simulink model "X_AXEmodel2"  (R2013b)
settings: Solver=ode45  StartTime=0.0  StopTime=10.0  RelTol=1e-3
libraries: simulink x3, arduinolib x2
settings Model: Creator=KOUSTA  LastModifiedBy=KOUSTA

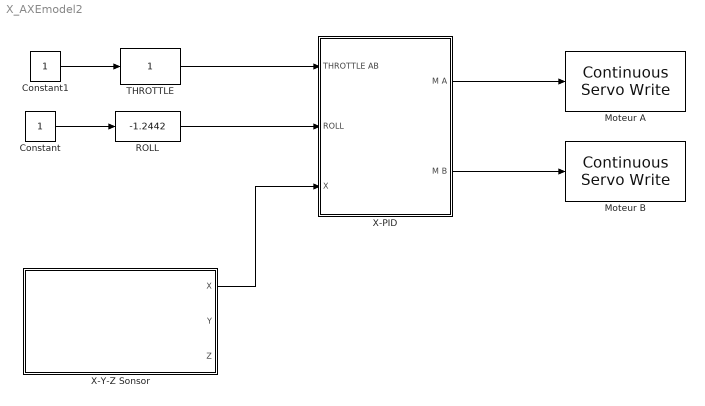
== system X_AXEmodel2 ==
  Constant : Constant
  Constant1 : Constant
  Moteur A : arduinolib/Continuous Servo Write  pinNumber=9
  Moteur B : arduinolib/Continuous Servo Write  pinNumber=3
  ROLL : simulink/Math Operations/Slider Gain  low=-90  gain=-1.2442  high=90
  THROTTLE : simulink/Math Operations/Slider Gain  low=0  gain=1  high=120
  X-PID : Subsystem
  X-Y-Z Sonsor : Subsystem
  wires:
  Constant/1 -> ROLL/1
  Constant1/1 -> THROTTLE/1
  ROLL/1 -> X-PID/2(ROLL)
  X-Y-Z Sonsor/1(X) -> X-PID/3(X)
  X-PID/1(M A) -> Moteur A/1
  X-PID/2(M B) -> Moteur B/1
  THROTTLE/1 -> X-PID/1(THROTTLE AB)

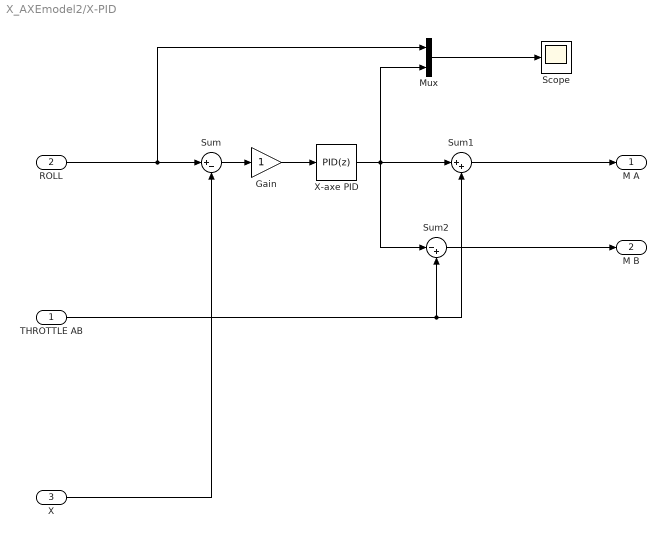
== system X_AXEmodel2/X-PID ==
  THROTTLE AB : Inport
  ROLL : Inport  Port=2
  X : Inport  Port=3
  Gain : Gain
  Mux : Mux  Inputs=2
  Scope : Scope
  Sum : Sum  Inputs=|+-
  Sum1 : Sum  Inputs=|++
  Sum2 : Sum  Inputs=|-+
  X-axe PID : simulink/Continuous/PID Controller  Controller=PID  TimeDomain=Discrete-time  SampleTime=1  IntegratorMethod=Forward Euler  FilterMethod=Forward Euler  Form=Parallel  P=1  I=1  D=0  N=100  InitialConditionSource=internal  InitialConditionForIntegrator=0  InitialConditionForFilter=0  ExternalReset=none  LimitOutput=off  UpperSaturationLimit=inf  LowerSaturationLimit=-inf  LinearizeAsGain=off  AntiWindupMode=none  Kb=1  TrackingMode=off  Kt=1  PParamMin=[]  PParamMax=[]  IParamMin=[]  IParamMax=[]  DParamMin=[]  DParamMax=[]  NParamMin=[]  NParamMax=[]  KbParamMin=[]  KbParamMax=[]  KtParamMin=[]  KtParamMax=[]  POutMin=[]  POutMax=[]  IOutMin=[]  IOutMax=[]  DOutMin=[]  DOutMax=[]  NOutMin=[]  NOutMax=[]  KbOutMin=[]  KbOutMax=[]  KtOutMin=[]  KtOutMax=[]  IntegratorOutMin=[]  IntegratorOutMax=[]  FilterOutMin=[]  FilterOutMax=[]  SumOutMin=[]  SumOutMax=[]  SumI1OutMin=[]  SumI1OutMax=[]  SumI2OutMin=[]  SumI2OutMax=[]  SumI3OutMin=[]  SumI3OutMax=[]  SumDOutMin=[]  SumDOutMax=[]  SaturationOutMin=[]  SaturationOutMax=[]  IntegratorContinuousStateAttributes=''  IntegratorStateMustResolveToSignalObject=off  IntegratorRTWStateStorageClass=Auto  FilterContinuousStateAttributes=''  FilterStateMustResolveToSignalObject=off  FilterRTWStateStorageClass=Auto
  M A : Outport
  M B : Outport  Port=2
  wires:
  Sum1/1 -> M A/1
  X-axe PID/1 -> Sum2/1, Mux/2, Sum1/1
  Sum2/1 -> M B/1
  X/1 -> Sum/2
  ROLL/1 -> Mux/1, Sum/1
  THROTTLE AB/1 -> Sum1/2, Sum2/2
  Mux/1 -> Scope/1
  Sum/1 -> Gain/1
  Gain/1 -> X-axe PID/1

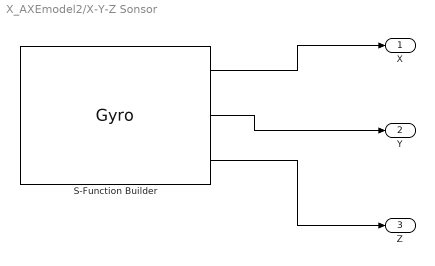
== system X_AXEmodel2/X-Y-Z Sonsor ==
  S-Function Builder : S-Function  InitFcn=try, set_param(gcb,'FunctionName','Gyro'), end  FunctionName=Gyro  SFunctionModules=Gyro_wrapper  EnableBusSupport=off  mask(S-Function Builder){}
      mask help: Simulink:masks:SFunctionBuilder_MD
      mask init:
      | val = [[.9  0.75 0.75 1 1 .9 .9 1]',[1 1 0.75 0.75 .9 .9 1 .9]'];try , sys = get_param(gcb,'SfunBuilderFcnName');if isempty(sys), sys = get_param(gcb,'FunctionName'); end,catch, sys = get_param(gcb,'FunctionName'); end
      settings: CopyFcn=set_param(gcbh,'LinkStatus','none')  PreSaveFcn=try, set_param(gcb,'FunctionName','Gyro'), end  OpenFcn=sfunctionwizard(gcbh)
      mask Display: plot(val(:,1),val(:,2)),disp(sys), port_label('output',1,'X'), port_label('output',2,'Y'), port_label('output',3,'Z')
  X : Outport
  Y : Outport  Port=2
  Z : Outport  Port=3
  wires:
  S-Function Builder/1 -> X/1
  S-Function Builder/2 -> Y/1
  S-Function Builder/3 -> Z/1
